simulink model "ship_Path_sin"  (Simulink 10.3)
settings: Solver=ode8  StartTime=0.0  StopTime=1000  FixedStep=0.1  RelTol=1e-3  EnableMultiTasking=on
libraries: simulink x1
settings Model: Creator=Administrator  LastModifiedBy=1179956468
settings DataIOCC: LimitDataPoints=on
settings DebuggingCC: SolverPrmCheckMsg=warning  FcnCallInpInsideContextMsg=error
settings ConfigComp: CovSFcnEnable=off

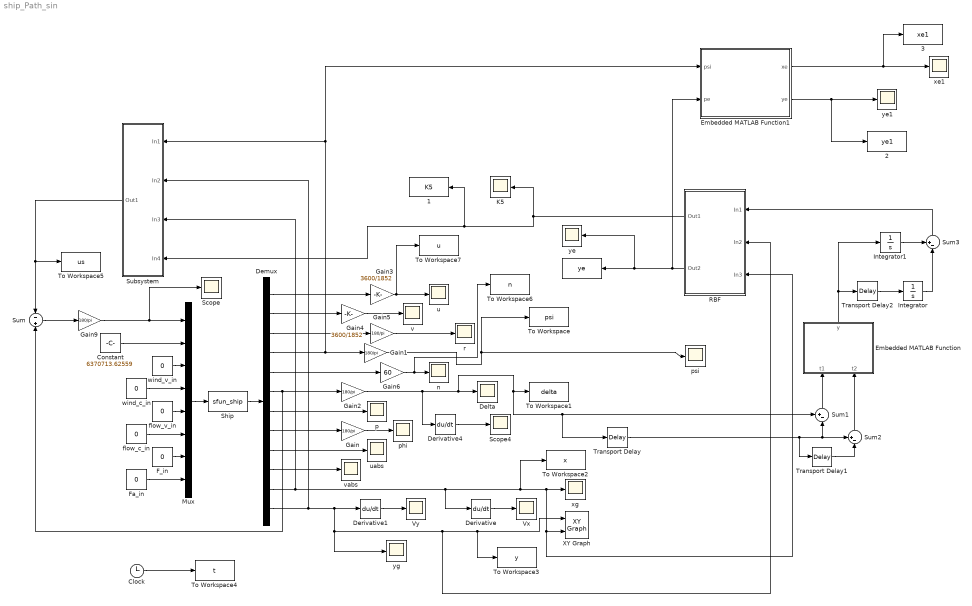
== system ship_Path_sin ==
  " " : ToWorkspace  VariableName=ye  SampleTime=-1
  " 1" : ToWorkspace  VariableName=K5  SampleTime=-1
  " 2" : ToWorkspace  VariableName=ye1  SampleTime=-1
  " 3" : ToWorkspace  VariableName=xe1  SampleTime=-1
  Clock : Clock
  Constant : Constant  Value=6370713.62559
  Delta : Scope
  Demux : Demux  Outputs=12
  Derivative : Derivative
  Derivative1 : Derivative
  Derivative4 : Derivative
  Embedded MATLAB Function : MATLAB Function  TreatAsAtomicUnit=on
  Embedded MATLAB Function1 : MATLAB Function  TreatAsAtomicUnit=on
  F_in : Constant  Value=0
  Fa_in : Constant  Value=0
  Gain{,1..2,5,9} (5 alike) : Gain  Gain=180/pi
  Gain3 : Gain  Gain=3600/1852
  Gain4 : Gain  Gain=3600/1852
  Gain6 : Gain  Gain=60
  Integrator : Integrator
  Integrator1 : Integrator
  K5 : Scope
  Mux : Mux  Inputs=8
  RBF : Subsystem
  Scope : Scope
  Scope4 : Scope
  Ship : S-Function  FunctionName=sfun_ship  SFunctionDeploymentMode=off  EnableBusSupport=off
  Subsystem : Subsystem
  Sum : Sum  Inputs=-|+
  Sum1 : Sum  Inputs=+-|
  Sum2 : Sum  Inputs=+-|
  Sum3 : Sum  Inputs=+-|
  To Workspace : ToWorkspace  VariableName=psi  SampleTime=-1
  To Workspace1 : ToWorkspace  VariableName=delta  SampleTime=-1
  To Workspace2 : ToWorkspace  VariableName=x  SampleTime=-1
  To Workspace3 : ToWorkspace  VariableName=y  SampleTime=-1
  To Workspace4 : ToWorkspace  VariableName=t  SampleTime=-1
  To Workspace5 : ToWorkspace  VariableName=us  SampleTime=-1
  To Workspace6 : ToWorkspace  VariableName=n  SampleTime=-1
  To Workspace7 : ToWorkspace  VariableName=u  SampleTime=-1
  Transport Delay : TransportDelay
  Transport Delay1 : TransportDelay
  Transport Delay2 : TransportDelay  DelayTime=50
  "Vx " : Scope
  Vy : Scope
  XY Graph : simulink/Sinks/XY Graph  xmin=-1000  xmax=14000  ymin=-800  ymax=500  st=-1
  flow_c_in : Constant  Value=0
  flow_v_in : Constant  Value=0
  n : Scope
  p : Scope
  phi : Scope
  psi : Scope
  r : Scope
  u : Scope
  uabs : Scope
  v : Scope
  vabs : Scope
  wind_c_in : Constant  Value=0
  wind_v_in : Constant  Value=0
  xe1 : Scope
  xg : Scope
  ye : Scope
  ye1 : Scope
  yg : Scope
  wires:
  Ship/1 -> Demux/1
  Demux/1 -> Gain3/1
  Demux/2 -> Gain4/1
  Demux/3 -> Gain5/1
  Demux/5 -> Gain6/1
  Demux/6 -> Sum/2, Gain2/1
  Demux/7 -> p/1
  Demux/8 -> Gain/1
  Gain/1 -> phi/1
  Gain3/1 -> u/1, To Workspace7/1
  Gain4/1 -> v/1
  Gain5/1 -> r/1
  Gain6/1 -> To Workspace6/1, n/1
  Demux/9 -> uabs/1
  Demux/10 -> vabs/1
  Demux/12 -> Derivative1/1, yg/1, XY Graph/1, To Workspace3/1, RBF/2(In2), Subsystem/2(In2)
  Demux/11 -> Derivative/1, xg/1, XY Graph/2, RBF/3(In3), To Workspace2/1, Subsystem/3(In3)
  Derivative/1 -> "Vx "/1
  Derivative1/1 -> Vy/1
  wind_v_in/1 -> Mux/3
  wind_c_in/1 -> Mux/4
  flow_v_in/1 -> Mux/5
  F_in/1 -> Mux/7
  Fa_in/1 -> Mux/8
  flow_c_in/1 -> Mux/6
  Mux/1 -> Ship/1
  Constant/1 -> Mux/2
  Sum/1 -> Gain9/1
  Derivative4/1 -> Scope4/1
  Subsystem/1(Out1) -> Sum/1, To Workspace5/1
  Demux/4 -> Gain1/1, Subsystem/1(In1), Embedded MATLAB Function1/1(psi)
  Gain2/1 -> Derivative4/1, Delta/1, To Workspace1/1, Sum1/1, Transport Delay/1
  Gain9/1 -> Mux/1, Scope/1
  Clock/1 -> To Workspace4/1
  Sum1/1 -> Embedded MATLAB Function/1(t1)
  Transport Delay1/1 -> Sum2/2
  Sum2/1 -> Embedded MATLAB Function/2(t2)
  Embedded MATLAB Function/1(y) -> Transport Delay2/1, Integrator1/1
  Transport Delay2/1 -> Integrator/1
  Integrator1/1 -> Sum3/1
  Integrator/1 -> Sum3/2
  Sum3/1 -> RBF/1(In1)
  RBF/1(Out1) -> Subsystem/4(In4), " 1"/1, K5/1
  Transport Delay/1 -> Transport Delay1/1, Sum1/2, Sum2/1
  RBF/2(Out2) -> Embedded MATLAB Function1/2(pe), " "/1, ye/1
  Embedded MATLAB Function1/2(ye) -> " 2"/1, ye1/1
  Embedded MATLAB Function1/1(xe) -> " 3"/1, xe1/1
  Gain1/1 -> psi/1, To Workspace/1

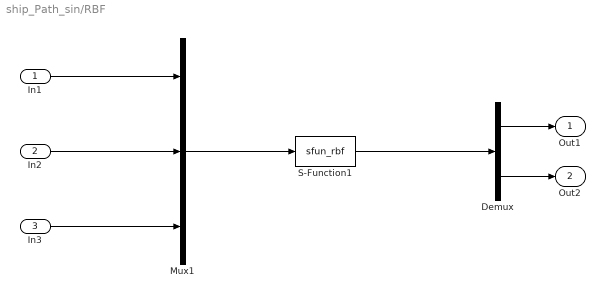
== system ship_Path_sin/RBF ==
  In1 : Inport
  In2 : Inport  Port=2
  In3 : Inport  Port=3
  Demux : Demux  Outputs=2
  Mux1 : Mux  Inputs=3
  S-Function1 : S-Function  FunctionName=sfun_rbf  SFunctionDeploymentMode=off  EnableBusSupport=off
  Out1 : Outport
  Out2 : Outport  Port=2
  wires:
  In1/1 -> Mux1/1
  In2/1 -> Mux1/2
  In3/1 -> Mux1/3
  Demux/1 -> Out1/1
  Demux/2 -> Out2/1
  Mux1/1 -> S-Function1/1
  S-Function1/1 -> Demux/1

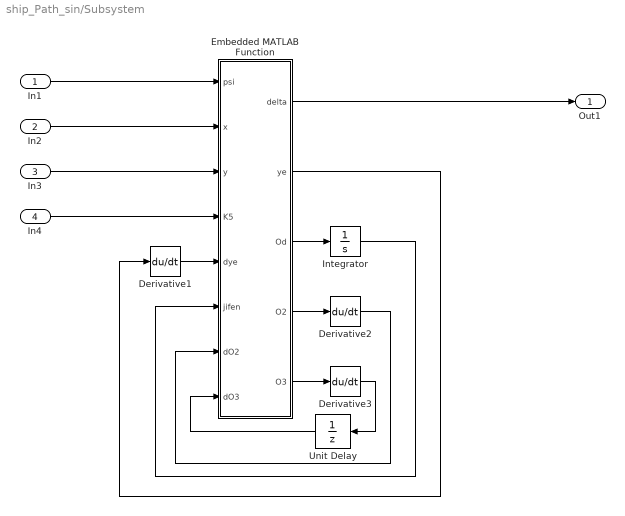
== system ship_Path_sin/Subsystem ==
  In1 : Inport
  In2 : Inport  Port=2
  In3 : Inport  Port=3
  In4 : Inport  Port=4
  Derivative1 : Derivative
  Derivative2 : Derivative
  Derivative3 : Derivative
  Embedded MATLAB Function : MATLAB Function  TreatAsAtomicUnit=on
  Integrator : Integrator
  Unit Delay : UnitDelay  SampleTime=-1  HasFrameUpgradeWarning=on
  Out1 : Outport
  wires:
  Embedded MATLAB Function/5(O3) -> Derivative3/1
  Derivative3/1 -> Unit Delay/1
  Embedded MATLAB Function/4(O2) -> Derivative2/1
  Derivative2/1 -> Embedded MATLAB Function/7(dO2)
  Integrator/1 -> Embedded MATLAB Function/6(jifen)
  Embedded MATLAB Function/1(delta) -> Out1/1
  Embedded MATLAB Function/3(Od) -> Integrator/1
  In1/1 -> Embedded MATLAB Function/1(psi)
  In2/1 -> Embedded MATLAB Function/2(x)
  In3/1 -> Embedded MATLAB Function/3(y)
  Embedded MATLAB Function/2(ye) -> Derivative1/1
  Derivative1/1 -> Embedded MATLAB Function/5(dye)
  Unit Delay/1 -> Embedded MATLAB Function/8(dO3)
  In4/1 -> Embedded MATLAB Function/4(K5)

== matlab function Embedded MATLAB Function ==
  data: t1 input double; y output double; t2 input double
function y = fcn(t1,t2)
% 滑模书式4.1.28 ,p为p_k(l)，
% y为式4.1.27的抖阵测量变量M的绝对值中的部分(未求和和绝对值)
% 输入舵角延迟t=1s（T=1仿真周期）
% simulink输出的y每50个控制周期累加一次输出(即y_jifen - y_delay50_jifen)即为M！！！！
if(t1*t2>0)
  p=0;
else
    p=1;
end
%y = p*abs(t1);%可以带绝对值也可以不带，舵角都很抖。。。。
y = p*t1;

== matlab function Subsystem/Embedded MATLAB Function ==
  data: psi input double; x input double; y input double; K5 input double; dye input double; delta output double; ye output double; Od output double; O2 output double; O3 output double; jifen input double; dO2 input double; dO3 input double
function [delta,ye,Od,O2,O3] = fcn(psi,x,y,K5, dye,jifen,dO2,dO3)
%K0=0.001;K1=10;K2=0.02;K3=0.011;K4=0.005;Te=2.5;%K5=13;
K0=0.000000001;K1=10;K2=1;K3=0.03;K4=0.01;Te=2.5;
ye=y-200*sin(pi*x/2500);%只跟踪ye，，路径跟踪的期望路径 yd=200*sin(pi*x/2500)，x为船舶实际x!!!!!!


O1=K1*f(K0*ye)+dye;%迭代滑模式4.1.10 ,zeta1(ye)即第一个滑模面
Od=f(O1);
O2=psi+K2*jifen;
O3=K3*f(O2)+dO2;
O4=K4*f(O3)+dO3;% 第四个滑模函数zeta4
%delta=-Te*K5*O4;% 滑模书式4.1.17(滑模面反馈率)和硕士论文式2.48(舵机特性)结合求得delta的微分
delta=Te*(-K5*O4-0.001*f(O4));% 应该是delta_E=delta+Te*d_delat(会发散)，为什么simulink用减号？？？
function mean=f(a)
mean=tanh(a);
% function mean=f(a)
% if(a<0.1&&a>-0.1)
%     mean=a;
% else 
%  mean=coth(a)-1/a;
% end

== matlab function Embedded MATLAB Function1 ==
  data: psi input double; xe output double; ye output double; pe input double
function [xe,ye] = fcn(psi,pe)
%#eml
xe=pe*cos(psi);
ye=pe*sin(psi);
